simulink model "L7_Project_207_1"  (R2023a)
settings: Solver=VariableStepAuto  StartTime=0.0  StopTime=3  RelTol=1e-3
libraries: slctrlblks x3, spsDCVoltageSourceLib x1, eeStairGenerator x1, spsPermanentMagnetSynchronousMachineLib x1, spsPWMGenerator2LevelLib x1, spsabctodq0Lib x1, spsdq0toabcLib x1, spsUniversalBridgeLib x1, sps_lib x1
settings Model: Creator=lipun  LastModifiedBy=lipun

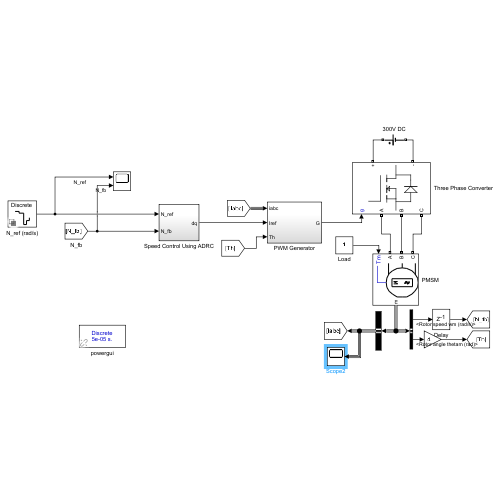
[thumbnail: Simulink's stored preview of the top-level diagram]
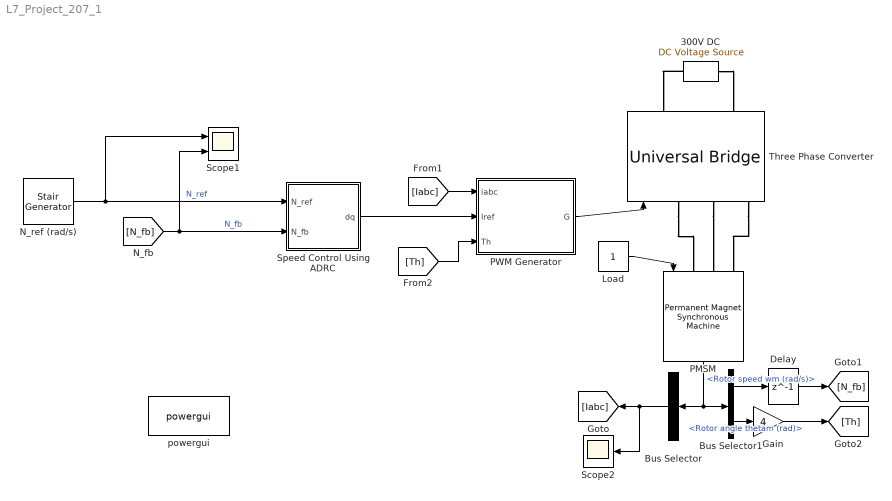
== system L7_Project_207_1 ==
  300V DC : spsDCVoltageSourceLib/DC Voltage Source  Amplitude=300  Measurements=None
  Bus Selector : BusSelector  OutputSignals=Stator current is_a (A),Stator current is_b (A),Stator current is_c (A)  OutputAsBus=on
  Bus Selector1 : BusSelector  OutputSignals=Rotor speed wm (rad/s),Rotor angle thetam (rad)
  Delay : Delay  DelayLength=1  InitialCondition=0  UseCircularBuffer=on
  Gain : Gain  Gain=4
  Load : Constant
  N_ref (rad/s) : eeStairGenerator/Stair Generator  LabelModeActiveChoice=Discrete  TimeInput=[0.2 0.9 1.6 2.1 2.6]  AmplitudeInput=[100 70 -100 -40 0]  SampleTime=-1  RepeatPattern=off  OutDataTypeStr=double
      settings: LibrarySourceBlock=ee_sl_lib/General Control/Stair Generator
  PMSM : spsPermanentMagnetSynchronousMachineLib/Permanent Magnet Synchronous Machine  NbPhases=3  FluxDistribution=Sinusoidal  RotorType=Salient-pole  MechanicalLoad=Torque Tm  PresetModel="07:  20 Nm 300 Vdc 2200 RPM - 33.9 Nm"  ShowDetailedParameters=on  MeasurementBus=off  Resistance=0.129  Inductance=8.5e-3  dqInductances=[0.001453 0.001607]  La=0.000395  MachineConstant=Flux linkage established by magnets (V.s)  Flux=0.1821  VoltageCst=132.1171  TorqueCst=1.0926  Flat=120  Mechanical=[0.003334 0.000425 4 0]  PolePairs=4  InitialConditions=[0,0, 0,0]  InitialConditions5ph=[0 0 0 0 0 0]  RefAngle=90 degrees behind phase A axis (modified Park)  IterativeDiscreteModel=Trapezoidal non iterative  TsBlock=-1  TsPowergui=0
  PWM Generator : Subsystem
  Scope1 : Scope  NumInputPorts=2
  Scope2 : Scope
  Speed Control Using ADRC : Subsystem
  Three Phase Converter : spsUniversalBridgeLib/Universal Bridge  Arms=3  SnubberResistance=10e5  SnubberCapacitance=inf  Device=MOSFET / Diodes  Ron=10e-3  Lon=0  ForwardVoltages="[  0  0  ]"  ForwardVoltage=0  GTOparameters=[ 10e-6 , 20e-6 ]  IGBTparameters=[ 1e-6 , 2e-6 ]  Measurements=None  Measurements_2=None  converterType=Rectifier
  powergui : sps_lib/powergui  Priority=1  SimulationMode=Discrete  SampleTime=50e-6  frequency=60  Iterations=50  frequencyindice=0  Pbase=100e6  ErrMax=1e-4  UnitsV=kV  UnitsW=MW  buscounter=0  FunctionMessages=off  echomessages=off  EnableUseOfTLC=off  CurrentSourceSwitches=off  DisableSnubberDevices=off  DisableRonSwitches=off  DisableVfSwitches=off  DisplayEquations=off  AutomaticDiscreteSolvers=off  SolverType=Tustin/Backward Euler (TBE)  Interpol=off  ExternalGateDelay=off  methode=off  Ts=100  x0status=blocks  SPID=on  SwTol=0  HookPort=off  NonlinearTolerance=1e-4  nMaxIteration=100  ContinueOnMaxIteration=off  RestoreLinks=warning  ResistiveCurrentMeasurement=off  Frange=[0:2:500]  Ylog=off  Xlog=on  ShowGrid=off  save=off  variable=ZData  structure=0  ZoomFFT=off  StartTime=0.0  cycles=1  DisplayStyle=1  fundamental=60  FreqAxis=off  MaxFrequency=1000  frequencyindicesteady=1  RmsSteady=1  display=off
  wires:
  N_ref (rad/s)/1 -> Scope1/1, Speed Control Using ADRC/1(N_ref)  "N_ref"
  Load/1 -> PMSM/1
  PWM Generator/1(G) -> Three Phase Converter/1
  [N_fb] -> Scope1/2, Speed Control Using ADRC/2(N_fb)  "N_fb"
  Delay/1 -> [N_fb]
  Bus Selector1/1 -> Delay/1  "<Rotor speed wm (rad/s)>"
  Gain/1 -> [Th]
  Bus Selector1/2 -> Gain/1  "<Rotor angle thetam (rad)>"
  Bus Selector/1 -> Scope2/1, [Iabc]
  [Th] -> PWM Generator/3(Th)
  [Iabc] -> PWM Generator/1(iabc)
  PMSM/1 -> Bus Selector1/1, Bus Selector/1
  Speed Control Using ADRC/1(dq) -> PWM Generator/2(Iref)
  connections:
  300V DC/RConn1 -- Three Phase Converter/RConn1
  300V DC/LConn1 -- Three Phase Converter/RConn2
  Three Phase Converter/LConn2 -- PMSM/LConn2
  Three Phase Converter/LConn3 -- PMSM/LConn3
  Three Phase Converter/LConn1 -- PMSM/LConn1

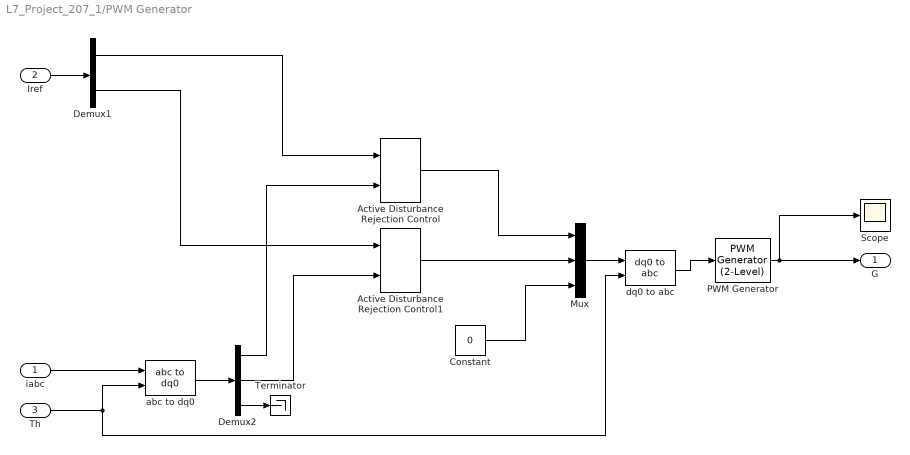
== system L7_Project_207_1/PWM Generator ==
  iabc : Inport
  Iref : Inport  Port=2
  Th : Inport  Port=3
  Active Disturbance Rejection Control : slctrlblks/Active Disturbance Rejection Control  time_domain=discrete-time  Ts=0.0001  model_type=second-order  b0=10  wc=1  wo=10  x0=0  ulim_checkbox=off  umax=inf  umin=-inf  xhat_checkbox=off
  Active Disturbance Rejection Control1 : slctrlblks/Active Disturbance Rejection Control  time_domain=discrete-time  Ts=0.0001  model_type=second-order  b0=10  wc=1  wo=10  x0=0  ulim_checkbox=off  umax=inf  umin=-inf  xhat_checkbox=off
  Constant : Constant  Value=0
  Demux1 : Demux  Outputs=2
  Demux2 : Demux  Outputs=3
  Mux : Mux  Inputs=3
  PWM Generator : spsPWMGenerator2LevelLib/PWM Generator (2-Level)  ModulatorType=Three-phase bridge (6 pulses)  ModulatorMode=Unsynchronized  Fc=27*60  Pc=90  nF=27  MinMax="[ -150  150 ]"  SamplingTechnique=Natural  ModulatingSignals=off  m=0.8  Freq=60  Phase=0  Ts=0  ShowCarrierOutport=off
  Scope : Scope
  Terminator : Terminator
  abc to dq0 : spsabctodq0Lib/abc to dq0  Alignment=90 degrees behind phase A axis
  dq0 to abc : spsdq0toabcLib/dq0 to abc  Alignment=90 degrees behind phase A axis
  G : Outport
  wires:
  Iref/1 -> Demux1/1
  Constant/1 -> Mux/3
  PWM Generator/1 -> Scope/1, G/1
  iabc/1 -> abc to dq0/1
  Th/1 -> dq0 to abc/2, abc to dq0/2
  abc to dq0/1 -> Demux2/1
  Demux2/3 -> Terminator/1
  Demux1/1 -> Active Disturbance Rejection Control/1
  Demux2/1 -> Active Disturbance Rejection Control/2
  Demux1/2 -> Active Disturbance Rejection Control1/1
  Demux2/2 -> Active Disturbance Rejection Control1/2
  dq0 to abc/1 -> PWM Generator/1
  Mux/1 -> dq0 to abc/1
  Active Disturbance Rejection Control/1 -> Mux/1
  Active Disturbance Rejection Control1/1 -> Mux/2

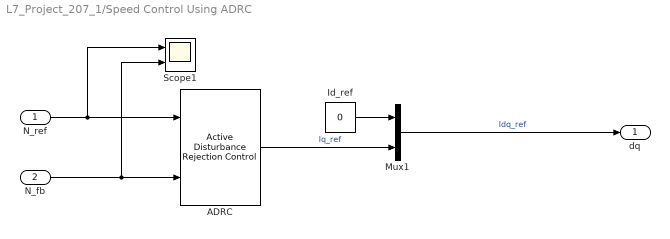
== system L7_Project_207_1/Speed Control Using ADRC ==
  N_ref : Inport
  N_fb : Inport  Port=2
  ADRC : slctrlblks/Active Disturbance Rejection Control  time_domain=discrete-time  Ts=0.00001  model_type=second-order  b0=1000  wc=455  wo=455*8  x0=0  ulim_checkbox=off  umax=inf  umin=-inf  xhat_checkbox=off
  Id_ref : Constant  Value=0
  Mux1 : Mux  Inputs=2
  Scope1 : Scope  NumInputPorts=2
  dq : Outport
  wires:
  Mux1/1 -> dq/1  "Idq_ref"
  Id_ref/1 -> Mux1/1
  ADRC/1 -> Mux1/2  "Iq_ref"
  N_ref/1 -> Scope1/1, ADRC/1
  N_fb/1 -> Scope1/2, ADRC/2
